simulink model "Terceroo"  (R2017b)
settings: Solver=VariableStepAuto  StartTime=0.0  StopTime=10.0  RelTol=1e-3
values from neighbouring files (symbols this model uses):
  kd = eval(S.kd)    [Cuarto_P_I_D.m]    (also in Quinto_P_I_D.m; Segundoo.m; SeptimoBPIDD2.m; SeptimoPIDD2.m)
  kp = eval(S.kp)    [Cuarto_P_I_D.m]    (also in Quinto_P_I_D.m; Segundoo.m; SeptimoBPIDD2.m; SeptimoPIDD2.m)
settings Model: Creator=Cx001la  LastModifiedBy=Cx001la

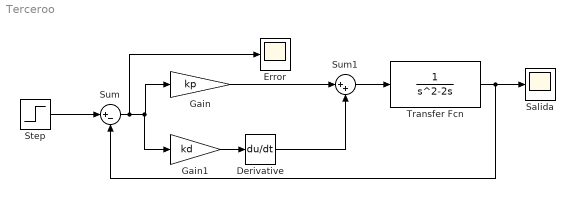
== system Terceroo ==
  Derivative : Derivative
  Error : Scope
  Gain : Gain  Gain=kp
  Gain1 : Gain  Gain=kd
  Salida : Scope
  Step : Step  Time=0  SampleTime=0
  Sum : Sum  Inputs=|+-
  Sum1 : Sum  Inputs=|++
  Transfer Fcn : TransferFcn  Denominator=[1 -2 0]
  wires:
  Step/1 -> Sum/1
  Sum/1 -> Error/1, Gain1/1, Gain/1
  Gain1/1 -> Derivative/1
  Derivative/1 -> Sum1/2
  Gain/1 -> Sum1/1
  Sum1/1 -> Transfer Fcn/1
  Transfer Fcn/1 -> Salida/1, Sum/2
